simulink model "magLev_sim"  (R2016b)
settings: Solver=ode4  StartTime=0.0  StopTime=T  FixedStep=ts  RelTol=1e-3
values from neighbouring files (symbols this model uses):
  GainScheduling = Simulink.Parameter(GainScheduling)    [main.m]    (also in main_GS.m)
  Gcs = ss(Ac,Bc,Cc,Dc, 'Name'     ,'PID', 'StateName',{'xc1','xc2','xc3'}, 'InputName',{'p'}, 'InputUnit',{'[m]'}, 'OutputName',{'V'}, 'OutputUnit',{'[Volt]'})    [main.m]
  sys = ss(A,B,C,D,      'name'     ,['Mag Lev trimmed p = ',num2str(position),' [m]'],      'StateName',{'p','v','i'},      'StateUnit',{'[m]','[m/s]','[A]'},      'InputName',{'V'},      'InputUnit',{'Volt'},      'OutputName',{'p'},      'OutputUnit',{'[m]'},      'UserData',trimPoint,      'Notes', [infoR,' | ',infoO])    [main.m]    (also in main_GS.m = ss(A,B,C,D,      'name'     ,['Mag Lev trimmed p = ',num2str)
  SystemCompensated = ss(Phi,G,H,L,      'name'     ,'Mag Lev + PID',      'StateName',{'p','v','i','xc1','xc2','xc3'},      'StateUnit',{'[m]','[m/s]','[A]','[m]','[m/s]','[m/s]'},      'InputName',{'p'},      'InputUnit',{'[p]'},      'OutputName',{'p','u'},      'OutputUnit',{'[m]','[V]'},      'UserData',trimPoint,      'Notes', [infoR,' | ',infoO])    [main.m]    (also in main_GS.m = ss(Phi,G,H,L,          'name'     ,'Mag Lev + LQI',         )
  trimPoint = struct    [main.m]
  ts = 0.01    [main.m]    (also in main_GS.m)
undefined symbols (not defined in the file or in its folder): A, B
settings Model: Creator=Gianni  LastModifiedBy=Gianni

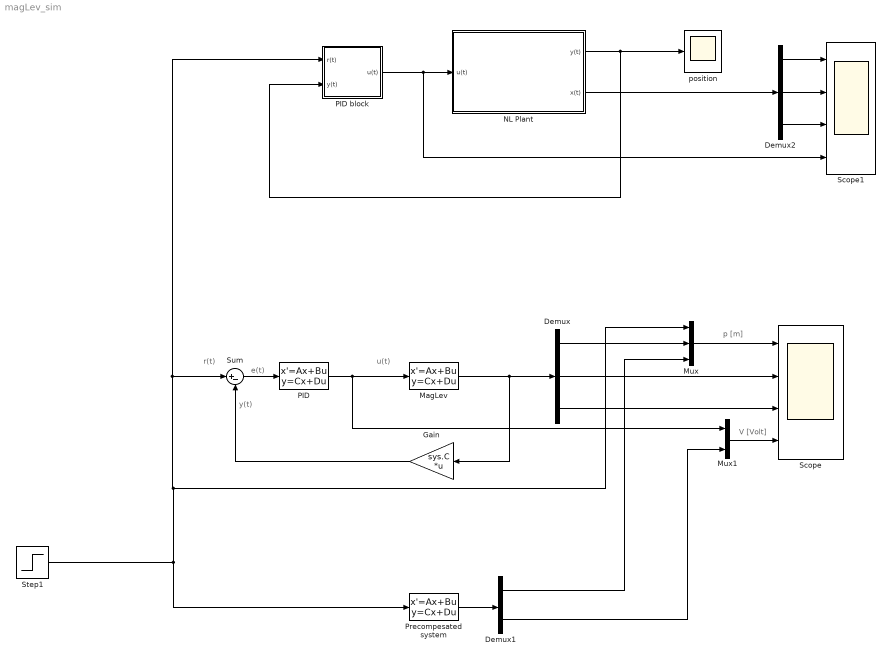
== system magLev_sim ==
  note: u(t)
  note: e(t)
  note: r(t)
  note: y(t)
  note: p [m]
  note: V [Volt]
  Demux : Demux  Outputs=3
  Demux1 : Demux  Outputs=2
  Demux2 : Demux  Outputs=3
  Gain : Gain  Gain=sys.C  Multiplication=Matrix(K*u)
  MagLev : StateSpace  A=sys.A  B=sys.B  C=eye(length(A))  D=zeros(size(B))  X0=0
  Mux : Mux  Inputs=3
  Mux1 : Mux  Inputs=2
  NL Plant : Subsystem
  PID : StateSpace  A=Gcs.A  B=Gcs.B  C=Gcs.C  D=Gcs.D  X0=0
  PID block : Subsystem
  Precompesated system : StateSpace  A=SystemCompensated.A  B=SystemCompensated.B  C=SystemCompensated.C  D=SystemCompensated.D  X0=0
  Scope : Scope  NumInputPorts=4
  Scope1 : Scope  NumInputPorts=4
  Step1 : Step  SampleTime=0
  Sum : Sum  Inputs=|+-
  position : Scope
  wires:
  PID/1 -> MagLev/1, Mux1/1
  MagLev/1 -> Gain/1, Demux/1
  Mux/1 -> Scope/1
  Demux/2 -> Scope/2
  Demux/3 -> Scope/3
  Mux1/1 -> Scope/4
  Precompesated system/1 -> Demux1/1
  Demux1/1 -> Mux/3
  Demux1/2 -> Mux1/2
  Sum/1 -> PID/1
  Demux/1 -> Mux/2
  Gain/1 -> Sum/2
  Demux2/1 -> Scope1/1
  Demux2/2 -> Scope1/2
  Demux2/3 -> Scope1/3
  NL Plant/2(x(t)) -> Demux2/1
  NL Plant/1(y(t)) -> PID block/2(y(t)), position/1
  Step1/1 -> Precompesated system/1, PID block/1(r(t)), Sum/1, Mux/1
  PID block/1(u(t)) -> Scope1/4, NL Plant/1(u(t))

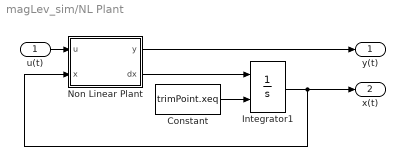
== system magLev_sim/NL Plant ==
  u(t) : Inport
  Constant : Constant  Value=trimPoint.xeq
  Integrator1 : Integrator  InitialConditionSource=external  InitialCondition=trimPoint.xeq
  Non Linear Plant : MATLAB Function  TreatAsAtomicUnit=on
  y(t) : Outport
  x(t) : Outport  Port=2
  wires:
  u(t)/1 -> Non Linear Plant/1(u)
  Non Linear Plant/1(y) -> y(t)/1
  Integrator1/1 -> x(t)/1, Non Linear Plant/2(x)
  Constant/1 -> Integrator1/2
  Non Linear Plant/2(dx) -> Integrator1/1

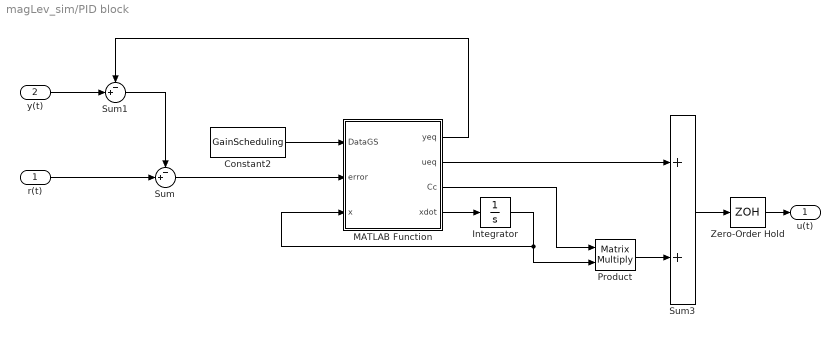
== system magLev_sim/PID block ==
  r(t) : Inport
  y(t) : Inport  Port=2
  Constant2 : Constant  Value=GainScheduling  OutDataTypeStr=Bus: GainSchedulingStruct
  Integrator : Integrator  InitialCondition=[0;0;0]
  MATLAB Function : MATLAB Function  TreatAsAtomicUnit=on
  Product : Product  Multiplication=Matrix(*)
  Sum : Sum  Inputs=-+|
  Sum1 : Sum  Inputs=-+|
  Sum3 : Sum
  Zero-Order Hold : ZeroOrderHold  SampleTime=ts
  u(t) : Outport
  wires:
  Sum3/1 -> Zero-Order Hold/1
  Constant2/1 -> MATLAB Function/1(DataGS)
  Zero-Order Hold/1 -> u(t)/1
  y(t)/1 -> Sum1/2
  Sum/1 -> MATLAB Function/2(error)
  MATLAB Function/4(xdot) -> Integrator/1
  Integrator/1 -> Product/2, MATLAB Function/3(x)
  MATLAB Function/2(ueq) -> Sum3/1
  MATLAB Function/1(yeq) -> Sum1/1
  r(t)/1 -> Sum/2
  Sum1/1 -> Sum/1
  Product/1 -> Sum3/2
  MATLAB Function/3(Cc) -> Product/1

== matlab function magLev_sim/PID block/MATLAB Function ==
  data: yeq output; ueq output; Cc output; DataGS input; xdot output; error input; x input
function [yeq,ueq,Cc,xdot] = PIDlogic(DataGS,error,x)
    ueq = DataGS.ueq;
    yeq = DataGS.yeq;
    
    Ac = DataGS.Ac;
    Bc = DataGS.Bc;
    Cc = DataGS.Cc;
    
    xdot = Ac*x + Bc*error;
    
end

== matlab function magLev_sim/NL Plant/Non Linear Plant ==
  data: u input; y output; x input; dx output
function [y,dx] = MagLev(u,x)

    g0 = 9.81;  R = 50;    L = 0.5;
    m  = 0.02; Km = 19.62; b = 0.1;
     
    x1 = x(1); % position [m]
    x2 = x(2); % velocity [m/s]
    x3 = x(3); % current  [A]

    %u % voltage  [V]

    dx = [x2;
          g0-(b/m)*x2-(Km/m)*((x3/x1)^2);
         (1/(L+Km/x1))*(-R*x3+Km*(x2/(x1^2))+u)];  
      y = x1;
end
